simulink model "fuzzy_logiz_control_first_Ke1_arxiko"  (R2019a)
settings: Solver=VariableStepAuto  StartTime=0.0  StopTime=10.0  RelTol=1e-3
values from neighbouring files (symbols this model uses):
  a = Ti    [Ergasia1_FuzzyControl.m]
  Ki = c*Kp    (= 3)    [Ergasia1_ClassicControl.m]
  Kp = 2.02913029039800    (= 2.0291302904)    [Ergasia1_ClassicControl.m]
libraries: simulink x1, fuzblock x1
settings Model: Creator=Konstantinos  LastModifiedBy=Konstantinos

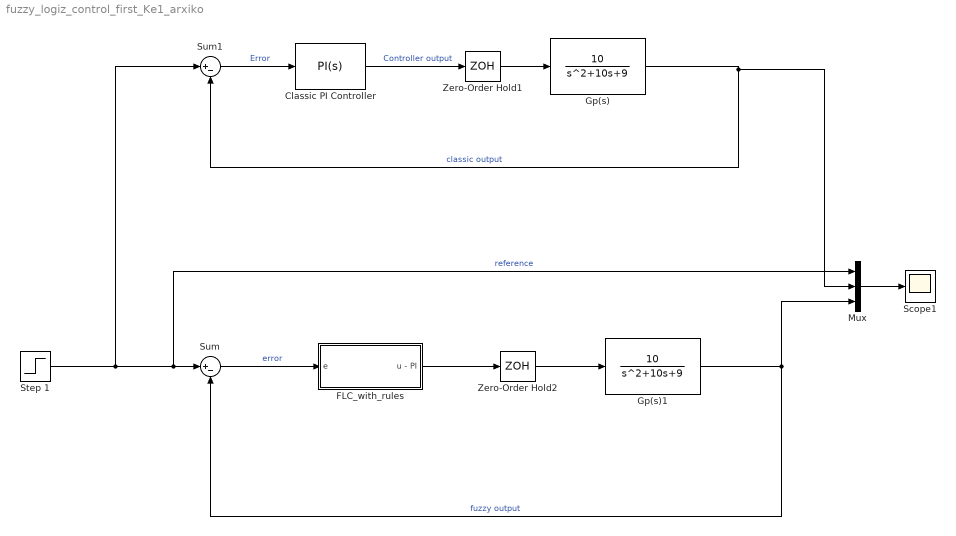
== system fuzzy_logiz_control_first_Ke1_arxiko ==
  Classic PI Controller : simulink/Continuous/PID Controller  Controller=PI  Form=Parallel  TimeDomain=Continuous-time  SampleTime=-1  IntegratorMethod=Forward Euler  FilterMethod=Forward Euler  ControllerParametersSource=internal  P=Kp  I=Ki  D=0.02  UseFilter=on  N=20  TunerSelectOption=Transfer Function Based (PID Tuner App)  InitialConditionSource=internal  InitialConditionForIntegrator=0  InitialConditionForFilter=0  DifferentiatorICPrevScaledInput=0  ExternalReset=none  TrackingMode=off  Kt=1  LimitOutput=off  UpperSaturationLimit=inf  LowerSaturationLimit=-inf  LinearizeAsGain=on  AntiWindupMode=none  Kb=1  POutMin=[]  POutMax=[]  IOutMin=[]  IOutMax=[]  DOutMin=[]  DOutMax=[]  NOutMin=[]  NOutMax=[]  SumOutMin=[]  SumOutMax=[]  SaturationOutMin=[]  SaturationOutMax=[]  PParamMin=[]  PParamMax=[]  IParamMin=[]  IParamMax=[]  DParamMin=[]  DParamMax=[]  NParamMin=[]  NParamMax=[]  KbParamMin=[]  KbParamMax=[]  KtParamMin=[]  KtParamMax=[]  KbOutMin=[]  KbOutMax=[]  KtOutMin=[]  KtOutMax=[]  IntegratorOutMin=[]  IntegratorOutMax=[]  FilterOutMin=[]  FilterOutMax=[]  SumI1OutMin=[]  SumI1OutMax=[]  SumI2OutMin=[]  SumI2OutMax=[]  SumI3OutMin=[]  SumI3OutMax=[]  SumI4OutMin=[]  SumI4OutMax=[]  SumDOutMin=[]  SumDOutMax=[]  DifferentiatorOutMin=[]  DifferentiatorOutMax=[]  FilterDiffOutCoefMin=[]  FilterDiffOutCoefMax=[]  ReciprocalOutMin=[]  ReciprocalOutMax=[]  SumDenOutMin=[]  SumDenOutMax=[]  SumNumOutMin=[]  SumNumOutMax=[]  DivideOutMin=[]  DivideOutMax=[]  IntegratorContinuousStateAttributes=''  IntegratorStateMustResolveToSignalObject=off  IntegratorRTWStateStorageClass=Auto  FilterContinuousStateAttributes=''  FilterStateMustResolveToSignalObject=off  FilterRTWStateStorageClass=Auto  ParallelPVariant=InternalParameters  IdealPVariant=Disabled  IVariant=InternalParameters  DVariant=Disabled  IntegratorVariant=Continuous  SatVariant=Disabled  AWVariant=Passthrough  PCopyVariant=Disabled  TRVariant=Disabled  FdbkBlocksVariant=Forward  IdealPFdbkVariant=Disabled  SatFdbkVariant=Disabled  DerivativeFilterVariant=Disabled  NVariant=Disabled  NCopyVariant=Disabled_SignalSpec  FilterICVariant=Disabled  IntegratorICVariant=InternalICs  ExternalResetVariant=Disabled  TRSumVariant=Passthrough  SumFdbkVariant=Disabled  SumVariant=Sum_PI
  FLC_with_rules : Subsystem
  Gp(s) : TransferFcn  Numerator=[10]  Denominator=[1 10 9]
  Gp(s)1 : TransferFcn  Numerator=[10]  Denominator=[1 10 9]
  Mux : Mux  Inputs=3
  Scope1 : Scope
  Step 1 : Step  Time=0  After=50  SampleTime=0.01
  Sum : Sum  Inputs=|+-
  Sum1 : Sum  Inputs=|+-
  Zero-Order Hold1 : ZeroOrderHold  SampleTime=0.01
  Zero-Order Hold2 : ZeroOrderHold  SampleTime=0.01
  wires:
  Gp(s)/1 -> Mux/2, Sum1/2  "classic output"
  Zero-Order Hold1/1 -> Gp(s)/1
  Sum1/1 -> Classic PI Controller/1  "Error"
  Classic PI Controller/1 -> Zero-Order Hold1/1  "Controller output"
  FLC_with_rules/1(u - PI) -> Zero-Order Hold2/1
  Zero-Order Hold2/1 -> Gp(s)1/1
  Sum/1 -> FLC_with_rules/1(e)  "error"
  Gp(s)1/1 -> Sum/2, Mux/3  "fuzzy output"
  Step 1/1 -> Sum1/1, Mux/1, Sum/1  "reference"
  Mux/1 -> Scope1/1

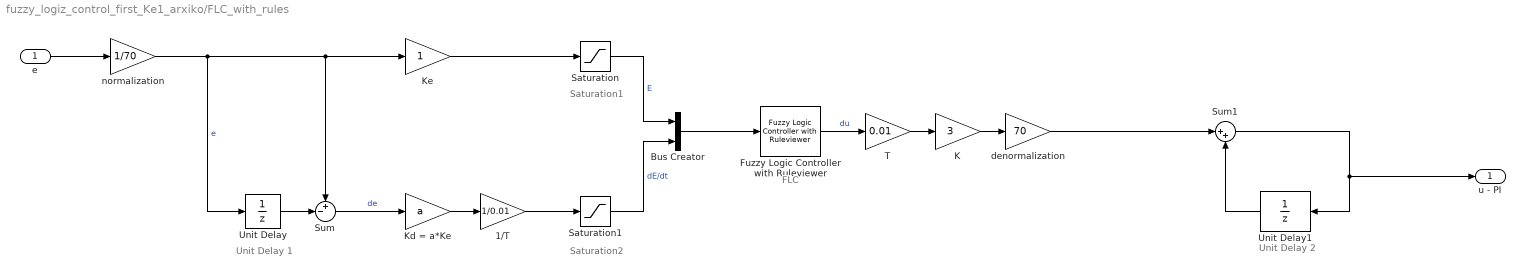
== system fuzzy_logiz_control_first_Ke1_arxiko/FLC_with_rules ==
  note: FLC
  note: Saturation2
  note: Saturation1
  note: Unit Delay 2
  note: Unit Delay 1
  e : Inport
  1/T : Gain  Gain=1/0.01
  Bus Creator : BusCreator  Inputs=2
  Fuzzy Logic Controller with Ruleviewer : fuzblock/Fuzzy Logic  Controller  with Ruleviewer  fismatrix=FLC_with_rules  Ts=0.01
  K : Gain  Gain=3
  Kd = a*Ke : Gain  Gain=a
  Ke : Gain
  Saturation : Saturate  UpperLimit=1  LowerLimit=-1
  Saturation1 : Saturate  UpperLimit=1  LowerLimit=-1
  Sum : Sum  Inputs=+-|
  Sum1 : Sum  Inputs=|++
  T : Gain  Gain=0.01
  Unit Delay : UnitDelay  SampleTime=-1  HasFrameUpgradeWarning=on
  Unit Delay1 : UnitDelay  SampleTime=-1  HasFrameUpgradeWarning=on
  denormalization : Gain  Gain=70
  normalization : Gain  Gain=1/70
  u - PI : Outport
  wires:
  Sum1/1 -> u - PI/1, Unit Delay1/1
  1/T/1 -> Saturation1/1
  Fuzzy Logic Controller with Ruleviewer/1 -> T/1  "du"
  denormalization/1 -> Sum1/1
  K/1 -> denormalization/1
  Saturation1/1 -> Bus Creator/2  "dE/dt"
  Saturation/1 -> Bus Creator/1  "E"
  Sum/1 -> Kd = a*Ke/1  "de"
  Unit Delay1/1 -> Sum1/2
  normalization/1 -> Ke/1, Sum/1, Unit Delay/1  "e"
  T/1 -> K/1
  Kd = a*Ke/1 -> 1/T/1
  Ke/1 -> Saturation/1
  Unit Delay/1 -> Sum/2
  e/1 -> normalization/1
  Bus Creator/1 -> Fuzzy Logic Controller with Ruleviewer/1
